simulink model "lab12_a"  (R2025b)
settings: Solver=ode45  StartTime=0  StopTime=3  RelTol=1e-3  EnableMultiTasking=on
undefined symbols (not defined in the file): index, k_feedforward, kp, kpi
libraries: simulink x1
settings Model: Creator=PC  LastModifiedBy=Lenovo
settings DataIOCC: SaveFormat=Array  SignalLoggingSaveFormat=ModelDataLogs  SignalLoggingName=sigsOut  ReturnWorkspaceOutputsName=SDOSimTest_Log
settings DebuggingCC: SaveWithParameterizedLinksMsg=none  UnderspecifiedInitializationDetection=Classic  MergeDetectMultiDrivingBlocksExec=none  SignalResolutionControl=TryResolveAllWithWarning  MultiTaskDSMMsg=warning  MultiTaskCondExecSysMsg=none  UnconnectedInputMsg=warning  UnconnectedOutputMsg=warning  UnconnectedLineMsg=warning
settings HardwareCC: ProdBitPerPointer=32.0  ProdBitPerSizeT=32.0  ProdBitPerPtrDiffT=32.0  ProdLargestAtomicFloat=None  ProdIntDivRoundTo=Undefined  ProdEndianess=Unspecified  ProdWordSize=32.0  ProdHWDeviceType=32-bit Generic  TargetUnknown=on
settings ModelReferenceCC: EnableRefExpFcnMdlSchedulingChecks=on  PropagateSignalLabelsOutOfModel=off
settings RTWCC: GPUComputeCapability=3.5  DLArmComputeVersion=19.05
settings GRTTargetCC: CombineOutputUpdateFcns=off  GRTInterface=on
settings ConfigComp: CovMetricSettings=dw  CovSaveCumulativeToWorkspaceVar=on  CovSaveSingleToWorkspaceVar=on

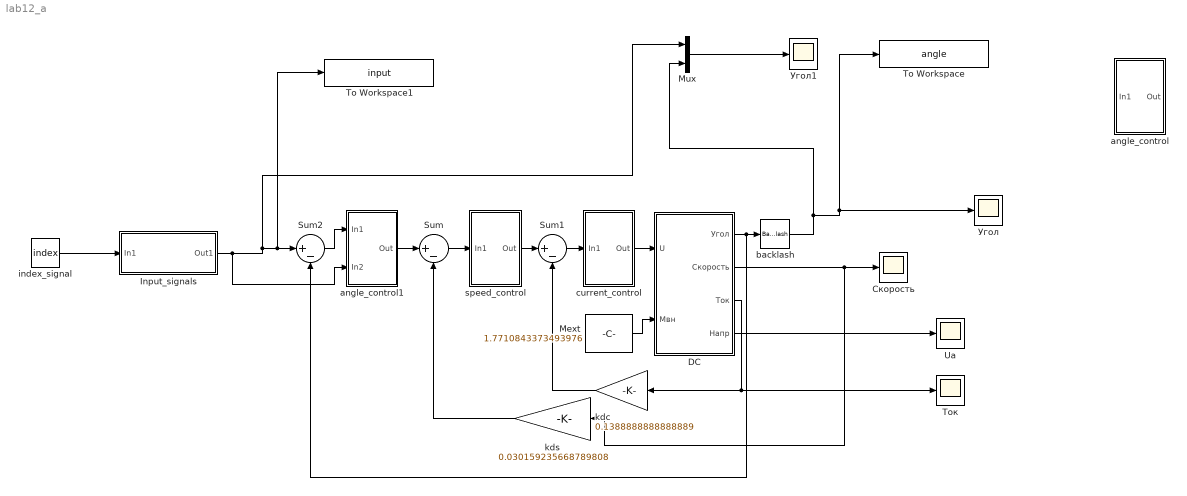
== system lab12_a ==
  DC : Subsystem
  Input_signals : Subsystem
  Mext : Constant  Value=1.7710843373493976
  Mux : Mux  Inputs=2
  Sum : Sum  Inputs=|+-  SaturateOnIntegerOverflow=on
  Sum1 : Sum  Inputs=|+-  SaturateOnIntegerOverflow=on
  Sum2 : Sum  Inputs=|+-  SaturateOnIntegerOverflow=on
  To Workspace : ToWorkspace  VariableName=angle  SaveFormat=Structure With Time  SampleTime=-1
  To Workspace1 : ToWorkspace  VariableName=input  SaveFormat=Structure With Time  SampleTime=-1
  Ua : Scope
      settings: SampleTime=0.001  TimeSpan=0.05353611419143481  ActiveDisplayYMinimum=-29.029207995662105  ActiveDisplayYMaximum=21.262871960959007  DataLoggingMaxPoints=50000  DataLoggingVariableName=ScopeData3
  angle_control : Subsystem
  angle_control1 : Subsystem
  backlash : Backlash  BacklashWidth=0.00029
  current_control : Subsystem
  index_signal : Constant  Value=index
  kdc : Gain  Gain=0.1388888888888889  SaturateOnIntegerOverflow=on  OutDataTypeStr=Inherit: Same as input  ParamDataTypeStr=Inherit: Same as input
  kds : Gain  Gain=0.030159235668789808  SaturateOnIntegerOverflow=on  OutDataTypeStr=Inherit: Same as input  ParamDataTypeStr=Inherit: Same as input
  speed_control : Subsystem
  Скорость : Scope
      settings: ActiveDisplayYMinimum=-1.8818916422998546  ActiveDisplayYMaximum=14.765924340526233  DataLoggingMaxPoints=50000
  Ток : Scope
      settings: SampleTime=0.00001  TimeSpan=0.5  ActiveDisplayYMinimum=-33.368370874163183  ActiveDisplayYMaximum=33.037145383700121  DataLoggingMaxPoints=50000  DataLoggingVariableName=ScopeData2
  Угол : Scope
      settings: SampleTime=0.001  ActiveDisplayYMinimum=-4.1597997421429218  ActiveDisplayYMaximum=37.438197679286304  DataLoggingMaxPoints=50000
  Угол1 : Scope
      settings: SampleTime=0.001  ActiveDisplayYMinimum=-1017.5162877725813  ActiveDisplayYMaximum=124.16847641917568  DataLoggingMaxPoints=50000  DataLoggingVariableName=ScopeData8
  wires:
  Mext/1 -> DC/2(Mвн)
  DC/2(Скорость) -> kds/1, Скорость/1
  DC/4(Напр) -> Ua/1
  Sum1/1 -> current_control/1(In1)
  DC/3(Ток) -> Ток/1, kdc/1
  kdc/1 -> Sum1/2
  kds/1 -> Sum/2
  DC/1(Угол) -> Sum2/2, backlash/1
  current_control/1(Out) -> DC/1(U)
  Sum/1 -> speed_control/1(In1)
  Mux/1 -> Угол1/1
  Input_signals/1(Out1) -> angle_control1/2(In2), Mux/1, To Workspace1/1, Sum2/1
  speed_control/1(Out) -> Sum1/1
  backlash/1 -> Mux/2, Угол/1, To Workspace/1
  angle_control1/1(Out) -> Sum/1
  Sum2/1 -> angle_control1/1(In1)
  index_signal/1 -> Input_signals/1(In1)

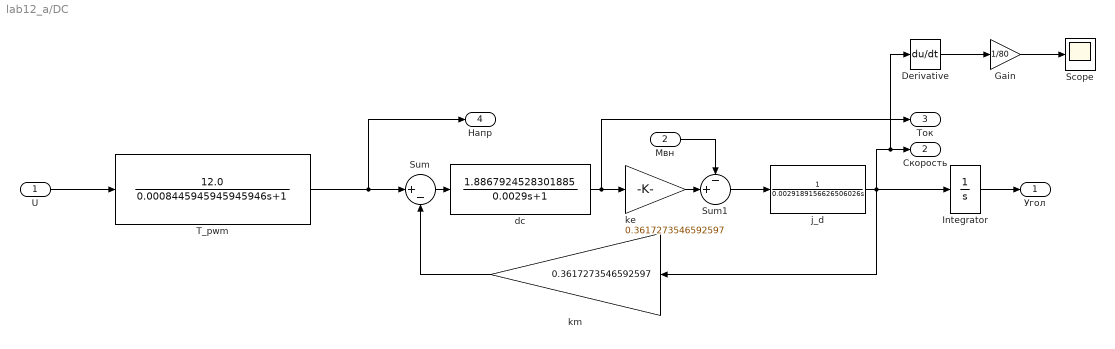
== system lab12_a/DC ==
  U : Inport
  Mвн : Inport  Port=2
  Derivative : Derivative
  Gain : Gain  Gain=1/80
  Integrator : Integrator
  Scope : Scope
      settings: ActiveDisplayYMinimum=-14.869427745911038  ActiveDisplayYMaximum=14.878639369679709  DataLoggingVariableName=ScopeData6
  Sum : Sum  Inputs=|+-  InputSameDT=on  SaturateOnIntegerOverflow=on  OutDataTypeStr=Inherit: Same as first input
  Sum1 : Sum  Inputs=-+|  InputSameDT=on  SaturateOnIntegerOverflow=on  OutDataTypeStr=Inherit: Same as first input
  T_pwm : TransferFcn  Numerator=12.0  Denominator=[0.0008445945945945946 1]
  dc : TransferFcn  Numerator=1.8867924528301885  Denominator=[0.0029 1]
  j_d : TransferFcn  Denominator=[0.0029189156626506026 0]
  ke : Gain  Gain=0.3617273546592597  SaturateOnIntegerOverflow=on  OutDataTypeStr=Inherit: Same as input  ParamDataTypeStr=Inherit: Same as input
  km : Gain  Gain=0.3617273546592597  SaturateOnIntegerOverflow=on  OutDataTypeStr=Inherit: Same as input  ParamDataTypeStr=Inherit: Same as input
  Угол : Outport
  Скорость : Outport  Port=2
  Ток : Outport  Port=3
  Напр : Outport  Port=4
  wires:
  Sum/1 -> dc/1
  Mвн/1 -> Sum1/1
  Sum1/1 -> j_d/1
  j_d/1 -> km/1, Derivative/1, Скорость/1, Integrator/1
  ke/1 -> Sum1/2
  Integrator/1 -> Угол/1
  U/1 -> T_pwm/1
  km/1 -> Sum/2
  dc/1 -> ke/1, Ток/1
  T_pwm/1 -> Напр/1, Sum/1
  Derivative/1 -> Gain/1
  Gain/1 -> Scope/1

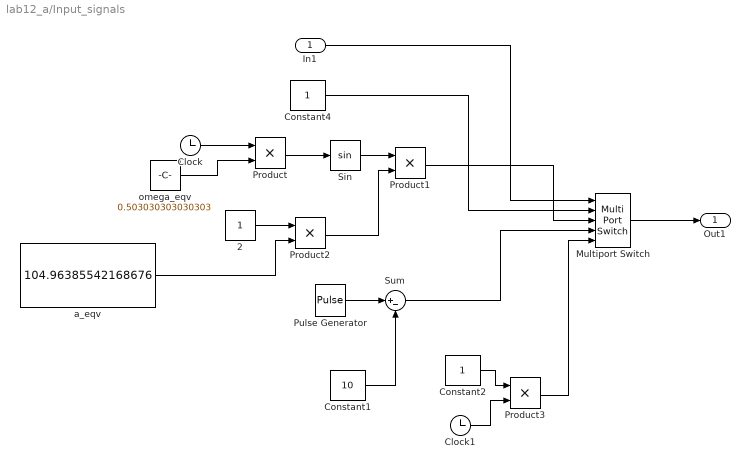
== system lab12_a/Input_signals ==
  In1 : Inport
  2 : Constant
  Clock : Clock
  Clock1 : Clock
  Constant1 : Constant  Value=10
  Constant2 : Constant
  Constant4 : Constant
  Multiport Switch : MultiPortSwitch  Inputs=4  SaturateOnIntegerOverflow=off  InputSameDT=off
  Product{,1..3} (4 alike) : Product
  Pulse Generator : DiscretePulseGenerator  PulseType=Time based  Amplitude=20  Period=1.5  PulseWidth=50
  Sin : Trigonometry
  Sum : Sum  Inputs=|+-
  a_eqv : Constant  Value=104.96385542168676
  omega_eqv : Constant  Value=0.503030303030303
  Out1 : Outport
  wires:
  2/1 -> Product2/1
  Product/1 -> Sin/1
  Product2/1 -> Product1/2
  Clock/1 -> Product/1
  omega_eqv/1 -> Product/2
  Sin/1 -> Product1/1
  Constant2/1 -> Product3/1
  a_eqv/1 -> Product2/2
  Clock1/1 -> Product3/2
  Multiport Switch/1 -> Out1/1
  In1/1 -> Multiport Switch/1
  Constant4/1 -> Multiport Switch/2
  Product1/1 -> Multiport Switch/3
  Pulse Generator/1 -> Sum/1
  Constant1/1 -> Sum/2
  Sum/1 -> Multiport Switch/4
  Product3/1 -> Multiport Switch/5

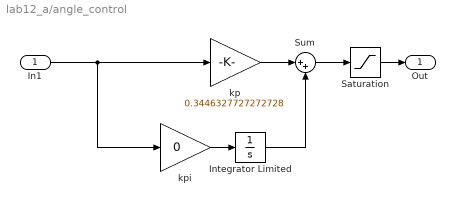
== system lab12_a/angle_control ==
  In1 : Inport
  Integrator Limited : Integrator  LimitOutput=on  UpperSaturationLimit=10  LowerSaturationLimit=-10
  Saturation : Saturate  UpperLimit=10  LowerLimit=-10
  Sum : Sum  Inputs=|++
  kp : Gain  Gain=0.3446327727272728  SaturateOnIntegerOverflow=on  OutDataTypeStr=Inherit: Same as input  ParamDataTypeStr=Inherit: Same as input
  kpi : Gain  Gain=0  SaturateOnIntegerOverflow=on  OutDataTypeStr=Inherit: Same as input  ParamDataTypeStr=Inherit: Same as input
  Out : Outport
  wires:
  In1/1 -> kpi/1, kp/1
  Saturation/1 -> Out/1
  kp/1 -> Sum/1
  Sum/1 -> Saturation/1
  kpi/1 -> Integrator Limited/1
  Integrator Limited/1 -> Sum/2

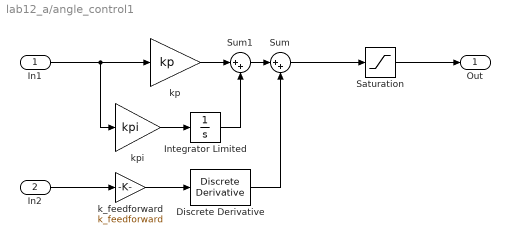
== system lab12_a/angle_control1 ==
  In1 : Inport
  In2 : Inport  Port=2
  Discrete Derivative : simulink/Quick Insert/Discrete/Discrete Derivative  gainval=1  ICPrevScaledInput=0.01  OutMin=[]  OutMax=[]  OutDataType=fixdt(1, 16)  OutScaling=2^-10  DoSatur=off
  Integrator Limited : Integrator  LimitOutput=on  UpperSaturationLimit=10  LowerSaturationLimit=-10
  Saturation : Saturate  UpperLimit=10  LowerLimit=-10
  Sum : Sum  Inputs=|++
  Sum1 : Sum  Inputs=|++
  k_feedforward : Gain  Gain=k_feedforward
  kp : Gain  Gain=kp  SaturateOnIntegerOverflow=on  OutDataTypeStr=Inherit: Same as input  ParamDataTypeStr=Inherit: Same as input
  kpi : Gain  Gain=kpi  SaturateOnIntegerOverflow=on  OutDataTypeStr=Inherit: Same as input  ParamDataTypeStr=Inherit: Same as input
  Out : Outport
  wires:
  Saturation/1 -> Out/1
  Integrator Limited/1 -> Sum1/2
  kpi/1 -> Integrator Limited/1
  kp/1 -> Sum1/1
  Sum1/1 -> Sum/1
  Sum/1 -> Saturation/1
  k_feedforward/1 -> Discrete Derivative/1
  In2/1 -> k_feedforward/1
  Discrete Derivative/1 -> Sum/2
  In1/1 -> kpi/1, kp/1

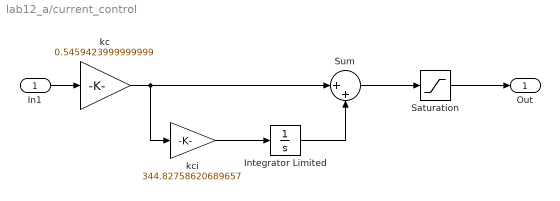
== system lab12_a/current_control ==
  In1 : Inport
  Integrator Limited : Integrator  LimitOutput=on  UpperSaturationLimit=10  LowerSaturationLimit=-10
  Saturation : Saturate  UpperLimit=10  LowerLimit=-10
  Sum : Sum  Inputs=|++  SaturateOnIntegerOverflow=on
  kc : Gain  Gain=0.5459423999999999  SaturateOnIntegerOverflow=on  OutDataTypeStr=Inherit: Same as input  ParamDataTypeStr=Inherit: Same as input
  kci : Gain  Gain=344.82758620689657  SaturateOnIntegerOverflow=on  OutDataTypeStr=Inherit: Same as input  ParamDataTypeStr=Inherit: Same as input
  Out : Outport
  wires:
  In1/1 -> kc/1
  kci/1 -> Integrator Limited/1
  Integrator Limited/1 -> Sum/2
  kc/1 -> Sum/1, kci/1
  Sum/1 -> Saturation/1
  Saturation/1 -> Out/1

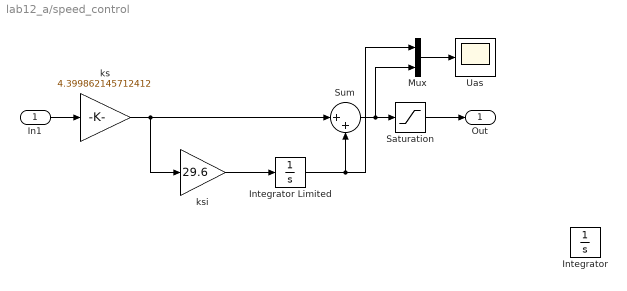
== system lab12_a/speed_control ==
  In1 : Inport
  Integrator : Integrator
  Integrator Limited : Integrator  LimitOutput=on  UpperSaturationLimit=10  LowerSaturationLimit=-10
  Mux : Mux  Inputs=2
  Saturation : Saturate  UpperLimit=10  LowerLimit=-10
  Sum : Sum  Inputs=|++  SaturateOnIntegerOverflow=on
  Uas : Scope
      settings: TimeSpan=0.05353611419143481  ActiveDisplayYMinimum=-1  ActiveDisplayYMaximum=1  DataLoggingMaxPoints=50000  DataLoggingVariableName=ScopeData5
  ks : Gain  Gain=4.399862145712412  SaturateOnIntegerOverflow=on  OutDataTypeStr=Inherit: Same as input  ParamDataTypeStr=Inherit: Same as input
  ksi : Gain  Gain=29.6  SaturateOnIntegerOverflow=on  OutDataTypeStr=Inherit: Same as input  ParamDataTypeStr=Inherit: Same as input
  Out : Outport
  wires:
  In1/1 -> ks/1
  ks/1 -> Sum/1, ksi/1
  Mux/1 -> Uas/1
  Integrator Limited/1 -> Sum/2, Mux/1
  ksi/1 -> Integrator Limited/1
  Sum/1 -> Saturation/1, Mux/2
  Saturation/1 -> Out/1
